simulink model "spring_mass_damper"  (R2024b)
settings: Solver=ode45  StartTime=0.0  StopTime=100  RelTol=1e-3
settings Model: Creator=kamimura  LastModifiedBy=kamimura

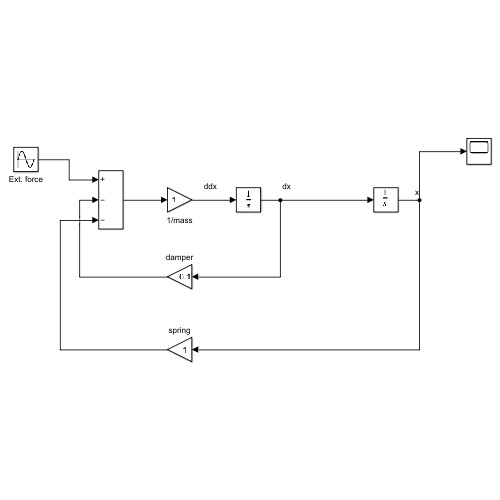
[thumbnail: Simulink's stored preview of the top-level diagram]
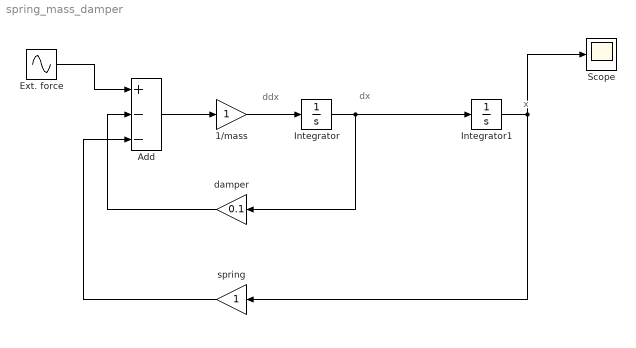
== system spring_mass_damper ==
  note: x
  note: ddx
  note: dx
  1/mass : Gain
  Add : Sum  Inputs=+--
  Ext. force : Sin  Amplitude=0.5  Frequency=0.5  SampleTime=0
  Integrator : Integrator
  Integrator1 : Integrator
  Scope : Scope
  damper : Gain  Gain=0.1
  spring : Gain
  wires:
  Add/1 -> 1/mass/1
  1/mass/1 -> Integrator/1
  Integrator/1 -> Integrator1/1, damper/1
  damper/1 -> Add/2
  Integrator1/1 -> spring/1, Scope/1
  spring/1 -> Add/3
  Ext. force/1 -> Add/1
